simulink model "midterm_sim"  (R2022b)
settings: Solver=VariableStepAuto  StartTime=0.0  StopTime=Tf  RelTol=1e-3
undefined symbols (not defined in the file): h0, J, kd_nonlin, kp_nonlin, mu, q_inertial2body_0, q_inertial2LVLH_0, q_LVLH2body_0, q_LVLH2body_f, r_inertial_0, rate_max, Tf_man, use_CMG, v_inertial_0, w_b_LVLH_man, w_body_wrt_inertial_0, w_LVLH_wrt_inertial_in_LVLH
libraries: matrix_library x2
settings Model: Creator=corey  LastModifiedBy=corey
settings DebuggingCC: UnconnectedInputMsg=warning  UnconnectedOutputMsg=warning  UnconnectedLineMsg=warning
settings ModelReferenceCC: EnableRefExpFcnMdlSchedulingChecks=on
settings RTWCC: DLArmComputeVersion=19.05

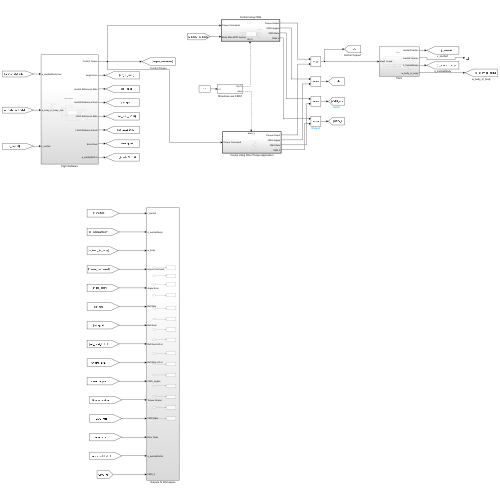
[thumbnail: Simulink's stored preview of the top-level diagram]
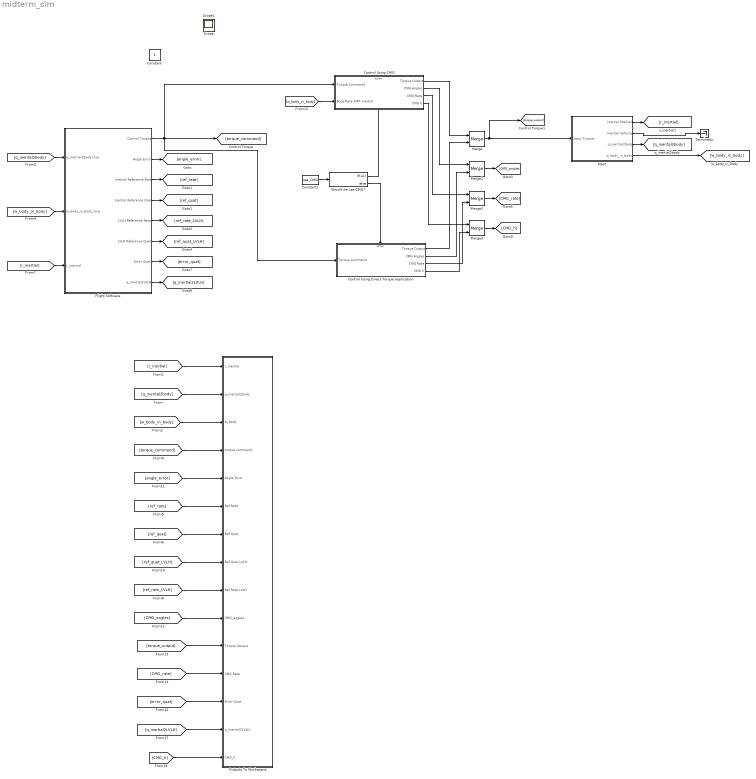
== system midterm_sim ==
  Constant1 : Constant  Value=use_CMG
  Control Using CMG : Subsystem  TreatAsAtomicUnit=on
  Control Using Direct Torque Application : Subsystem  TreatAsAtomicUnit=on
  Flight Software : Subsystem
  Merge{,1..3} (4 alike) : Merge
  Outputs To Workspace : Subsystem
  Plant : Subsystem
  Should we use CMG? : If  IfExpression=u1
  Terminator : Terminator
  Constant : Constant  IOType=siggen
  Scope : Scope
  Scope1 : Scope
  wires:
  Plant/4(w_body_in_body) -> [w_body_in_body]
  Plant/3(q_inertial2body) -> [q_inerital2body]
  Plant/2(Inertial Velocity) -> Terminator/1
  Plant/1(Inertial Position) -> [r_inertial]
  [q_inerital2body] -> Outputs To Workspace/2(q_inertial2body)
  [w_body_in_body] -> Outputs To Workspace/3(w_body)
  [r_inertial] -> Outputs To Workspace/1(r_inertial)
  [torque_command] -> Outputs To Workspace/4(torque command)
  Flight Software/1(Control Torque) -> Control Using CMG/1(Torque Command), Control Using Direct Torque Application/1(Torque Command), [torque_command]
  [angle_error] -> Outputs To Workspace/5(Angle Error)
  Flight Software/2(Angle Error) -> [angle_error]
  [q_inerital2body] -> Flight Software/1(q_inertial2body true)
  [w_body_in_body] -> Flight Software/2(w_body_in_body_true)
  Flight Software/3(Inertial Reference Rate) -> [ref_rate]
  Flight Software/4(Inertial Reference Quat) -> [ref_quat]
  [ref_rate] -> Outputs To Workspace/6(Ref Rate)
  [ref_quat] -> Outputs To Workspace/7(Ref Quat)
  [ref_rate_LVLH] -> Outputs To Workspace/9(Ref Rate LVLH)
  [ref_quat_LVLH] -> Outputs To Workspace/8(Ref Quat LVLH)
  Flight Software/5(LVLH Reference Rate) -> [ref_rate_LVLH]
  Flight Software/6(LVLH Reference Quat) -> [ref_quat_LVLH]
  [r_inertial] -> Flight Software/3(r_inertial)
  [CMG_angles] -> Outputs To Workspace/10(CMG_angles)
  [torque_output] -> Outputs To Workspace/11(Torque Output)
  [CMG_rate] -> Outputs To Workspace/12(CMG Rate)
  Constant1/1 -> Should we use CMG?/1
  Should we use CMG?/1 -> Control Using CMG/Action
  Should we use CMG?/2 -> Control Using Direct Torque Application/Action
  Control Using CMG/1(Torque Output) -> Merge/1
  Control Using Direct Torque Application/1(Torque Output) -> Merge/2
  Control Using CMG/2(CMG Angles) -> Merge1/1
  Control Using Direct Torque Application/2(CMG Angles) -> Merge1/2
  Control Using CMG/3(CMG Rate) -> Merge2/1
  Control Using Direct Torque Application/3(CMG Rate) -> Merge2/2
  Merge/1 -> Plant/1(Input Torque), [torque_output]
  Merge1/1 -> [CMG_angles]
  Merge2/1 -> [CMG_rate]
  [w_body_in_body] -> Control Using CMG/2(Body Rate WRT Inertial)
  Flight Software/7(Error Quat) -> [error_quat]
  [error_quat] -> Outputs To Workspace/13(Error Quat)
  Flight Software/8(q_inertial2LVLH) -> [q_inertial2LVLH]
  [q_inertial2LVLH] -> Outputs To Workspace/14(q_inertial2LVLH)
  Merge3/1 -> [CMG_h]
  Control Using CMG/4(CMG h) -> Merge3/1
  Control Using Direct Torque Application/4(CMG h) -> Merge3/2
  [CMG_h] -> Outputs To Workspace/15(CMG_h)

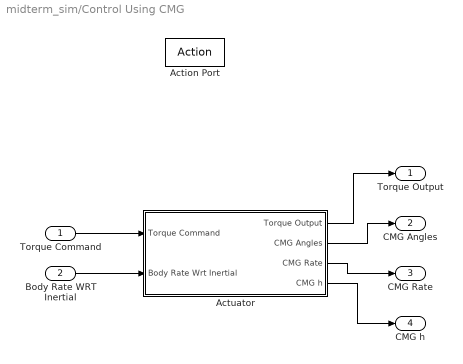
== system midterm_sim/Control Using CMG ==
  Torque Command : Inport
  Body Rate WRT Inertial : Inport  Port=2
  Action Port : ActionPort  ActionPortLabel=if(u1)
  Actuator : Subsystem
  Torque Output : Outport
  CMG Angles : Outport  Port=2
  CMG Rate : Outport  Port=3
  CMG h : Outport  Port=4
  wires:
  Torque Command/1 -> Actuator/1(Torque Command)
  Body Rate WRT Inertial/1 -> Actuator/2(Body Rate Wrt Inertial)
  Actuator/1(Torque Output) -> Torque Output/1
  Actuator/2(CMG Angles) -> CMG Angles/1
  Actuator/3(CMG Rate) -> CMG Rate/1
  Actuator/4(CMG h) -> CMG h/1

== system midterm_sim/Control Using Direct Torque Application ==
  Torque Command : Inport
  Action Port : ActionPort  ActionPortLabel=else
  Constant : Constant  Value=[0 0 0 0 0 0 0 0]'
  Constant1 : Constant  Value=[0 0 0]'
  Torque Output : Outport
  CMG Angles : Outport  Port=2
  CMG Rate : Outport  Port=3
  CMG h : Outport  Port=4
  wires:
  Constant/1 -> CMG Angles/1, CMG Rate/1
  Torque Command/1 -> Torque Output/1
  Constant1/1 -> CMG h/1

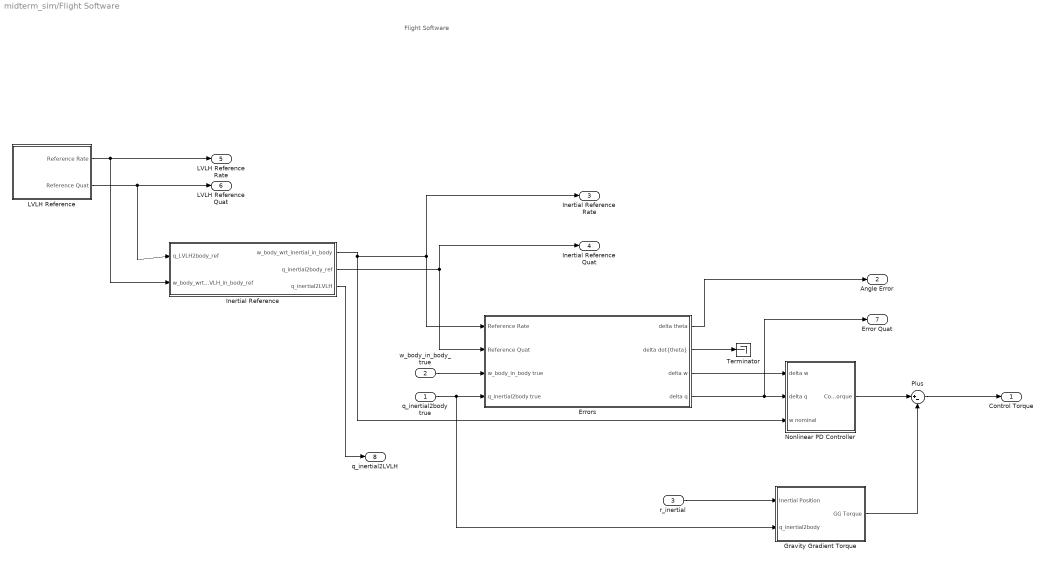
== system midterm_sim/Flight Software ==
  note: Flight Software
  q_inertial2body true : Inport
  w_body_in_body_true : Inport  Port=2
  r_inertial : Inport  Port=3
  Errors : Subsystem
  Gravity Gradient Torque : Subsystem
  Inertial Reference : Subsystem
  LVLH Reference : Subsystem
  Nonlinear PD Controller : Subsystem
  Plus : Sum  Inputs=|+-
  Terminator : Terminator
  Control Torque : Outport
  Angle Error : Outport  Port=2
  Inertial Reference Rate : Outport  Port=3
  Inertial Reference Quat : Outport  Port=4
  LVLH Reference Rate : Outport  Port=5
  LVLH Reference Quat : Outport  Port=6
  Error Quat : Outport  Port=7
  q_inertial2LVLH : Outport  Port=8
  wires:
  Errors/1(delta theta) -> Angle Error/1
  q_inertial2body true/1 -> Gravity Gradient Torque/2(q_inertial2body), Errors/4(q_inertial2body true)
  w_body_in_body_true/1 -> Errors/3(w_body_in_body true)
  Inertial Reference/1(w_body_wrt_inertial_in_body) -> Nonlinear PD Controller/3(w nominal), Inertial Reference Rate/1, Errors/1(Reference Rate)
  Inertial Reference/2(q_inertial2body_ref) -> Errors/2(Reference Quat), Inertial Reference Quat/1
  LVLH Reference/1(Reference Rate) -> Inertial Reference/2(w_body_wrt_LVLH_in_body_ref), LVLH Reference Rate/1
  LVLH Reference/2(Reference Quat) -> Inertial Reference/1(q_LVLH2body_ref), LVLH Reference Quat/1
  Errors/3(delta w) -> Nonlinear PD Controller/1(delta w)
  Errors/4(delta q) -> Error Quat/1, Nonlinear PD Controller/2(delta q)
  Errors/2("delta dot{theta}") -> Terminator/1
  Nonlinear PD Controller/1(Control Torque) -> Plus/1
  Plus/1 -> Control Torque/1
  Gravity Gradient Torque/1(GG Torque) -> Plus/2
  r_inertial/1 -> Gravity Gradient Torque/1(Inertial Position)
  Inertial Reference/3(q_inertial2LVLH) -> q_inertial2LVLH/1

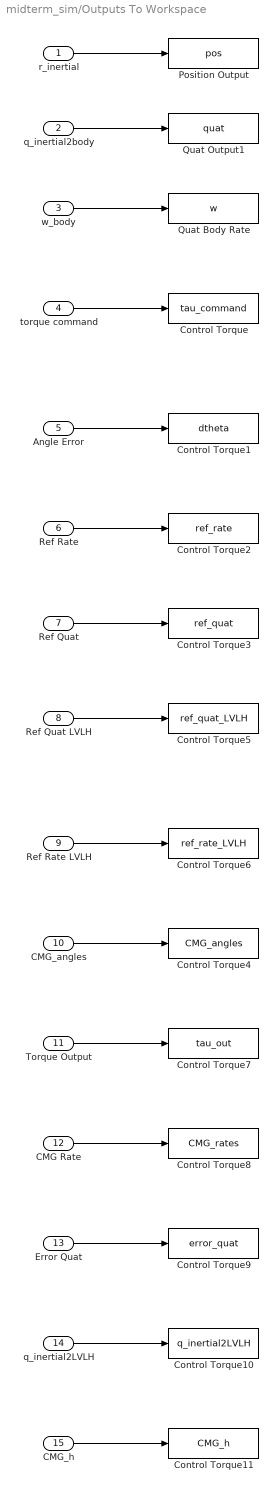
== system midterm_sim/Outputs To Workspace ==
  r_inertial : Inport
  q_inertial2body : Inport  Port=2
  w_body : Inport  Port=3
  torque command : Inport  Port=4
  Angle Error : Inport  Port=5
  Ref Rate : Inport  Port=6
  Ref Quat : Inport  Port=7
  Ref Quat LVLH : Inport  Port=8
  Ref Rate LVLH : Inport  Port=9
  CMG_angles : Inport  Port=10
  Torque Output : Inport  Port=11
  CMG Rate : Inport  Port=12
  Error Quat : Inport  Port=13
  q_inertial2LVLH : Inport  Port=14
  CMG_h : Inport  Port=15
  Control Torque : ToWorkspace  VariableName=tau_command  SampleTime=-1
  Control Torque1 : ToWorkspace  VariableName=dtheta  SampleTime=-1
  Control Torque10 : ToWorkspace  VariableName=q_inertial2LVLH  SampleTime=-1
  Control Torque11 : ToWorkspace  VariableName=CMG_h  SampleTime=-1
  Control Torque2 : ToWorkspace  VariableName=ref_rate  SampleTime=-1
  Control Torque3 : ToWorkspace  VariableName=ref_quat  SampleTime=-1
  Control Torque4 : ToWorkspace  VariableName=CMG_angles  SampleTime=-1
  Control Torque5 : ToWorkspace  VariableName=ref_quat_LVLH  SampleTime=-1
  Control Torque6 : ToWorkspace  VariableName=ref_rate_LVLH  SampleTime=-1
  Control Torque7 : ToWorkspace  VariableName=tau_out  SampleTime=-1
  Control Torque8 : ToWorkspace  VariableName=CMG_rates  SampleTime=-1
  Control Torque9 : ToWorkspace  VariableName=error_quat  SampleTime=-1
  Position Output : ToWorkspace  VariableName=pos  SampleTime=-1
  Quat Body Rate : ToWorkspace  VariableName=w  SampleTime=-1
  Quat Output1 : ToWorkspace  VariableName=quat  SampleTime=-1
  wires:
  r_inertial/1 -> Position Output/1
  w_body/1 -> Quat Body Rate/1
  q_inertial2body/1 -> Quat Output1/1
  torque command/1 -> Control Torque/1
  Angle Error/1 -> Control Torque1/1
  Ref Rate/1 -> Control Torque2/1
  Ref Quat/1 -> Control Torque3/1
  Ref Quat LVLH/1 -> Control Torque5/1
  Ref Rate LVLH/1 -> Control Torque6/1
  CMG_angles/1 -> Control Torque4/1
  Torque Output/1 -> Control Torque7/1
  CMG Rate/1 -> Control Torque8/1
  Error Quat/1 -> Control Torque9/1
  q_inertial2LVLH/1 -> Control Torque10/1
  CMG_h/1 -> Control Torque11/1

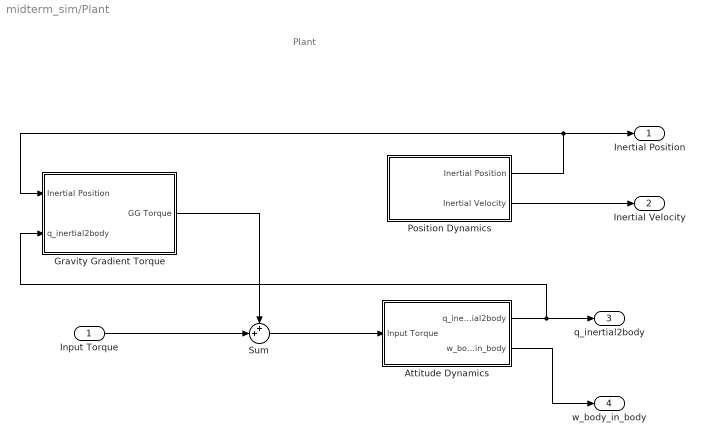
== system midterm_sim/Plant ==
  note: Plant
  Input Torque : Inport
  Attitude Dynamics : Subsystem
  Gravity Gradient Torque : Subsystem
  Position Dynamics : Subsystem
  Sum : Sum  Inputs=++|
  Inertial Position : Outport
  Inertial Velocity : Outport  Port=2
  q_inertial2body : Outport  Port=3
  w_body_in_body : Outport  Port=4
  wires:
  Position Dynamics/1(Inertial Position) -> Gravity Gradient Torque/1(Inertial Position), Inertial Position/1
  Position Dynamics/2(Inertial Velocity) -> Inertial Velocity/1
  Attitude Dynamics/1(q_inertial2body) -> Gravity Gradient Torque/2(q_inertial2body), q_inertial2body/1
  Attitude Dynamics/2(w_body_in_body) -> w_body_in_body/1
  Input Torque/1 -> Sum/2
  Sum/1 -> Attitude Dynamics/1(Input Torque)
  Gravity Gradient Torque/1(GG Torque) -> Sum/1

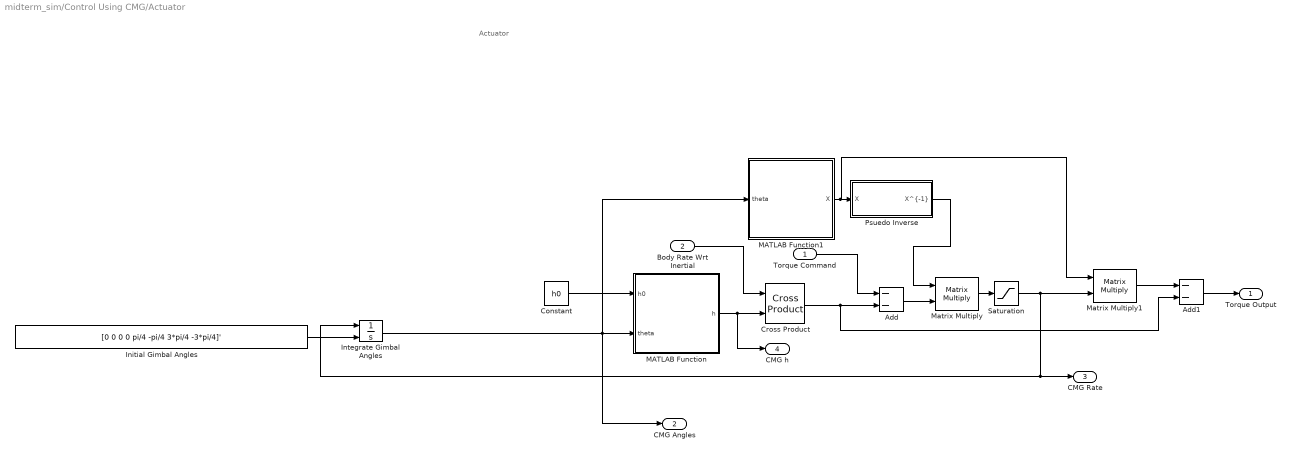
== system midterm_sim/Control Using CMG/Actuator ==
  note: Actuator
  Torque Command : Inport
  Body Rate Wrt Inertial : Inport  Port=2
  Add : Sum  Inputs=--
  Add1 : Sum  Inputs=--
  Constant : Constant  Value=h0
  Cross Product : matrix_library/Cross Product
  Initial Gimbal Angles : Constant  Value=[0 0 0 0 pi/4 -pi/4 3*pi/4 -3*pi/4]'
  Integrate Gimbal Angles : Integrator  InitialConditionSource=external
  MATLAB Function : MATLAB Function  TreatAsAtomicUnit=on
  MATLAB Function1 : MATLAB Function  TreatAsAtomicUnit=on
  Matrix Multiply : Product  Multiplication=Matrix(*)
  Matrix Multiply1 : Product  Multiplication=Matrix(*)
  Psuedo Inverse : Subsystem
  Saturation : Saturate  UpperLimit=rate_max  LowerLimit=-1*rate_max
  Torque Output : Outport
  CMG Angles : Outport  Port=2
  CMG Rate : Outport  Port=3
  CMG h : Outport  Port=4
  wires:
  Initial Gimbal Angles/1 -> Integrate Gimbal Angles/2
  Constant/1 -> MATLAB Function/1(h0)
  Cross Product/1 -> Add1/2, Add/2
  Torque Command/1 -> Add/1
  Body Rate Wrt Inertial/1 -> Cross Product/1
  MATLAB Function/1(h) -> CMG h/1, Cross Product/2
  MATLAB Function1/1(X) -> Matrix Multiply1/1, Psuedo Inverse/1(X)
  Psuedo Inverse/1("X^{-1}") -> Matrix Multiply/1
  Add/1 -> Matrix Multiply/2
  Matrix Multiply1/1 -> Add1/1
  Add1/1 -> Torque Output/1
  Integrate Gimbal Angles/1 -> MATLAB Function/2(theta), CMG Angles/1, MATLAB Function1/1(theta)
  Matrix Multiply/1 -> Saturation/1
  Saturation/1 -> Integrate Gimbal Angles/1, CMG Rate/1, Matrix Multiply1/2

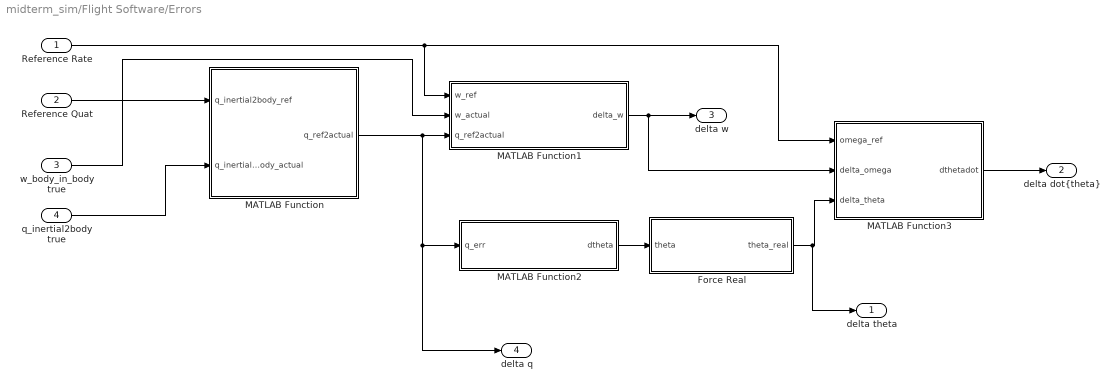
== system midterm_sim/Flight Software/Errors ==
  Reference Rate : Inport
  Reference Quat : Inport  Port=2
  w_body_in_body true : Inport  Port=3
  q_inertial2body true : Inport  Port=4
  Force Real : MATLAB Function  TreatAsAtomicUnit=on
  MATLAB Function : MATLAB Function  TreatAsAtomicUnit=on
  MATLAB Function1 : MATLAB Function  TreatAsAtomicUnit=on
  MATLAB Function2 : MATLAB Function  TreatAsAtomicUnit=on
  MATLAB Function3 : MATLAB Function  TreatAsAtomicUnit=on
  delta theta : Outport
  "delta dot{theta}" : Outport  Port=2
  delta w : Outport  Port=3
  delta q : Outport  Port=4
  wires:
  Reference Quat/1 -> MATLAB Function/1(q_inertial2body_ref)
  q_inertial2body true/1 -> MATLAB Function/2(q_inertial2body_actual)
  MATLAB Function/1(q_ref2actual) -> delta q/1, MATLAB Function2/1(q_err), MATLAB Function1/3(q_ref2actual)
  Reference Rate/1 -> MATLAB Function3/1(omega_ref), MATLAB Function1/1(w_ref)
  w_body_in_body true/1 -> MATLAB Function1/2(w_actual)
  MATLAB Function3/1(dthetadot) -> "delta dot{theta}"/1
  MATLAB Function2/1(dtheta) -> Force Real/1(theta)
  Force Real/1(theta_real) -> delta theta/1, MATLAB Function3/3(delta_theta)
  MATLAB Function1/1(delta_w) -> delta w/1, MATLAB Function3/2(delta_omega)

== system midterm_sim/Flight Software/Gravity Gradient Torque ==
  Inertial Position : Inport
  q_inertial2body : Inport  Port=2
  GG Torque Computation : MATLAB Function  TreatAsAtomicUnit=on
  Gravity Constant : Constant  Value=mu
  Inerita Matrix : Constant  Value=J
  MATLAB Function : MATLAB Function  TreatAsAtomicUnit=on
  GG Torque : Outport
  wires:
  Inerita Matrix/1 -> GG Torque Computation/1(J)
  Inertial Position/1 -> MATLAB Function/2(r), GG Torque Computation/3(r_inertial)
  q_inertial2body/1 -> GG Torque Computation/4(q_inertial2body)
  GG Torque Computation/1(T) -> GG Torque/1
  Gravity Constant/1 -> MATLAB Function/1(mu)
  MATLAB Function/1(n) -> GG Torque Computation/2(n)

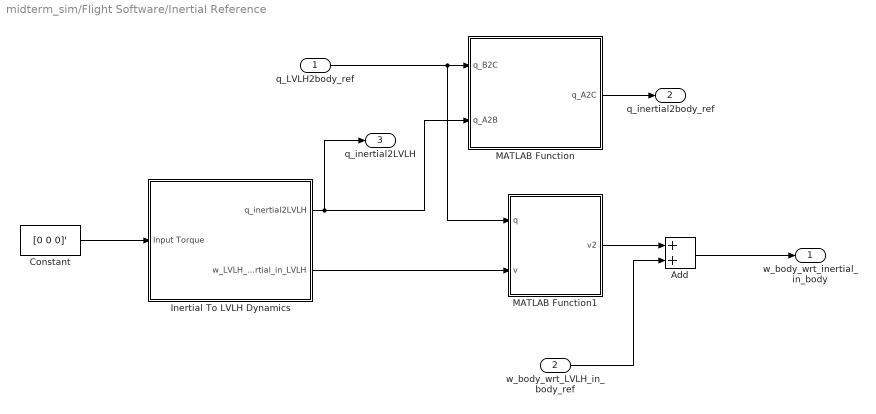
== system midterm_sim/Flight Software/Inertial Reference ==
  q_LVLH2body_ref : Inport
  w_body_wrt_LVLH_in_body_ref : Inport  Port=2
  Add : Sum
  Constant : Constant  Value=[0 0 0]'
  Inertial To LVLH Dynamics : Subsystem
  MATLAB Function : MATLAB Function  TreatAsAtomicUnit=on
  MATLAB Function1 : MATLAB Function  TreatAsAtomicUnit=on
  w_body_wrt_inertial_in_body : Outport
  q_inertial2body_ref : Outport  Port=2
  q_inertial2LVLH : Outport  Port=3
  wires:
  Constant/1 -> Inertial To LVLH Dynamics/1(Input Torque)
  Inertial To LVLH Dynamics/1(q_inertial2LVLH) -> MATLAB Function/2(q_A2B), q_inertial2LVLH/1
  MATLAB Function/1(q_A2C) -> q_inertial2body_ref/1
  q_LVLH2body_ref/1 -> MATLAB Function1/1(q), MATLAB Function/1(q_B2C)
  Inertial To LVLH Dynamics/2(w_LVLH_wrt_inertial_in_LVLH) -> MATLAB Function1/2(v)
  MATLAB Function1/1(v2) -> Add/1
  Add/1 -> w_body_wrt_inertial_in_body/1
  w_body_wrt_LVLH_in_body_ref/1 -> Add/2

== system midterm_sim/Flight Software/LVLH Reference ==
  Attitude Hold : Subsystem  TreatAsAtomicUnit=on
  Attitude Slew : Subsystem  TreatAsAtomicUnit=on
  Clock : Clock
  If : If  IfExpression=u1 < Tf_man
  Merge : Merge
  Merge1 : Merge
  Reference Rate : Outport
  Reference Quat : Outport  Port=2
  wires:
  Clock/1 -> If/1
  If/1 -> Attitude Slew/Action
  If/2 -> Attitude Hold/Action
  Attitude Slew/1(q_LVLH2body) -> Merge/1
  Attitude Hold/1(q_inertial2body) -> Merge/2
  Merge/1 -> Reference Quat/1
  Merge1/1 -> Reference Rate/1
  Attitude Slew/2(w_body_in_body) -> Merge1/1
  Attitude Hold/2(w_body) -> Merge1/2

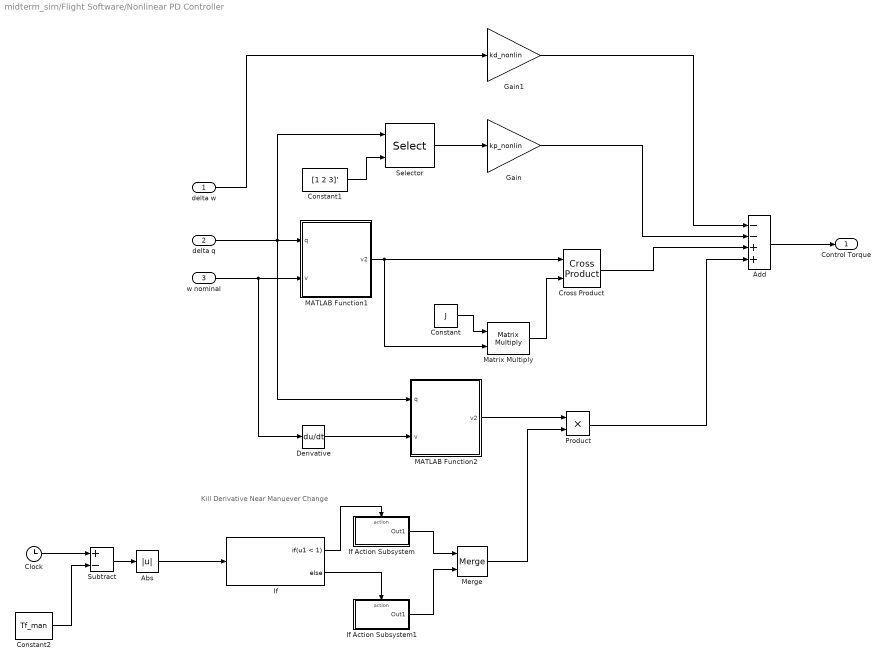
== system midterm_sim/Flight Software/Nonlinear PD Controller ==
  note: Kill Derivative Near Manuever Change
  delta w : Inport
  delta q : Inport  Port=2
  w nominal : Inport  Port=3
  Abs : Abs  SaturateOnIntegerOverflow=off
  Add : Sum  Inputs=--++
  Clock : Clock
  Constant : Constant  Value=J
  Constant1 : Constant  Value=[1 2 3]'
  Constant2 : Constant  Value=Tf_man
  Cross Product : matrix_library/Cross Product
  Derivative : Derivative  CoefficientInTFapproximation=Inf
  Gain : Gain  Gain=kp_nonlin
  Gain1 : Gain  Gain=kd_nonlin
  If : If  IfExpression=u1 < 1
  If Action Subsystem : Subsystem  TreatAsAtomicUnit=on
  If Action Subsystem1 : Subsystem  TreatAsAtomicUnit=on
  MATLAB Function1 : MATLAB Function  TreatAsAtomicUnit=on
  MATLAB Function2 : MATLAB Function  TreatAsAtomicUnit=on
  Matrix Multiply : Product  Multiplication=Matrix(*)
  Merge : Merge
  Product : Product
  Selector : Selector  InputPortWidth=4  IndexOptions=Index vector (port)  Indices=[1 3]  OutputSizes=1
  Subtract : Sum  Inputs=+-
  Control Torque : Outport
  wires:
  delta q/1 -> Selector/1, MATLAB Function2/1(q), MATLAB Function1/1(q)
  w nominal/1 -> Derivative/1, MATLAB Function1/2(v)
  MATLAB Function1/1(v2) -> Matrix Multiply/2, Cross Product/1
  Constant/1 -> Matrix Multiply/1
  Matrix Multiply/1 -> Cross Product/2
  Derivative/1 -> MATLAB Function2/2(v)
  Add/1 -> Control Torque/1
  Constant1/1 -> Selector/2
  Selector/1 -> Gain/1
  Gain/1 -> Add/2
  delta w/1 -> Gain1/1
  Gain1/1 -> Add/1
  MATLAB Function2/1(v2) -> Product/1
  Product/1 -> Add/4
  Cross Product/1 -> Add/3
  If/1 -> If Action Subsystem/Action
  If/2 -> If Action Subsystem1/Action
  Clock/1 -> Subtract/1
  Constant2/1 -> Subtract/2
  Subtract/1 -> Abs/1
  Abs/1 -> If/1
  If Action Subsystem/1(Out1) -> Merge/1
  If Action Subsystem1/1(Out1) -> Merge/2
  Merge/1 -> Product/2

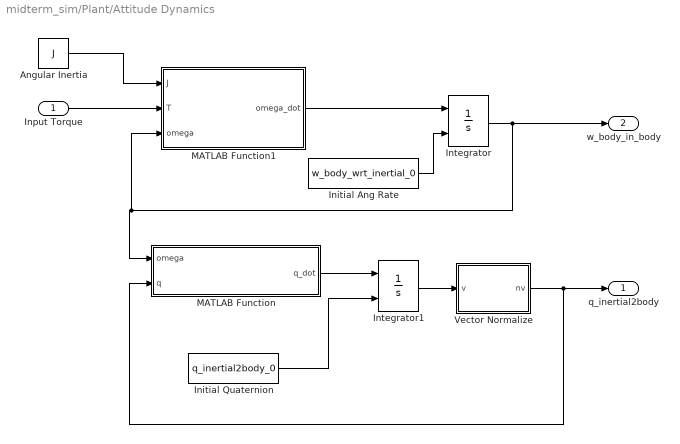
== system midterm_sim/Plant/Attitude Dynamics ==
  Input Torque : Inport
  Angular Inertia : Constant  Value=J
  Initial Ang Rate : Constant  Value=w_body_wrt_inertial_0
  Initial Quaternion : Constant  Value=q_inertial2body_0
  Integrator : Integrator  InitialConditionSource=external
  Integrator1 : Integrator  InitialConditionSource=external
  MATLAB Function : MATLAB Function  TreatAsAtomicUnit=on
  MATLAB Function1 : MATLAB Function  TreatAsAtomicUnit=on
  Vector Normalize : MATLAB Function  TreatAsAtomicUnit=on
  q_inertial2body : Outport
  w_body_in_body : Outport  Port=2
  wires:
  Integrator/1 -> MATLAB Function1/3(omega), MATLAB Function/1(omega), w_body_in_body/1
  MATLAB Function1/1(omega_dot) -> Integrator/1
  Initial Ang Rate/1 -> Integrator/2
  MATLAB Function/1(q_dot) -> Integrator1/1
  Initial Quaternion/1 -> Integrator1/2
  Integrator1/1 -> Vector Normalize/1(v)
  Vector Normalize/1(nv) -> MATLAB Function/2(q), q_inertial2body/1
  Input Torque/1 -> MATLAB Function1/2(T)
  Angular Inertia/1 -> MATLAB Function1/1(J)

== system midterm_sim/Plant/Gravity Gradient Torque ==
  Inertial Position : Inport
  q_inertial2body : Inport  Port=2
  GG Torque Computation : MATLAB Function  TreatAsAtomicUnit=on
  Gravity Constant : Constant  Value=mu
  Inerita Matrix : Constant  Value=J
  MATLAB Function : MATLAB Function  TreatAsAtomicUnit=on
  GG Torque : Outport
  wires:
  Inerita Matrix/1 -> GG Torque Computation/1(J)
  Inertial Position/1 -> MATLAB Function/2(r), GG Torque Computation/3(r_inertial)
  q_inertial2body/1 -> GG Torque Computation/4(q_inertial2body)
  GG Torque Computation/1(T) -> GG Torque/1
  Gravity Constant/1 -> MATLAB Function/1(mu)
  MATLAB Function/1(n) -> GG Torque Computation/2(n)

== system midterm_sim/Plant/Position Dynamics ==
  Gravity Constant : Constant  Value=mu
  Initial Position : Constant  Value=r_inertial_0
  Initial Velocity : Constant  Value=v_inertial_0
  Integrator : Integrator  InitialConditionSource=external  InitialCondition=[6871, 0, 0]'
  Integrator1 : Integrator  InitialConditionSource=external  InitialCondition=[0, 7.6166, 0]'
  Vector Norm : MATLAB Function  TreatAsAtomicUnit=on
  Inertial Position : Outport
  Inertial Velocity : Outport  Port=2
  wires:
  Integrator/1 -> Vector Norm/1(r), Inertial Position/1  "Position"
  Integrator1/1 -> Inertial Velocity/1, Integrator/1  "Velocity"
  Vector Norm/1(a) -> Integrator1/1  "Accel"
  Gravity Constant/1 -> Vector Norm/2(mu)
  Initial Velocity/1 -> Integrator1/2
  Initial Position/1 -> Integrator/2

== system midterm_sim/Control Using CMG/Actuator/Psuedo Inverse ==
  X : Inport
  Matrix Divide : Product  Inputs=*/  Multiplication=Matrix(*)
  Matrix Multiply : Product  Multiplication=Matrix(*)
  Transpose : Math  Operator=transpose
  "X^{-1}" : Outport
  wires:
  Transpose/1 -> Matrix Divide/1, Matrix Multiply/2
  X/1 -> Transpose/1, Matrix Multiply/1
  Matrix Multiply/1 -> Matrix Divide/2
  Matrix Divide/1 -> "X^{-1}"/1

== system midterm_sim/Flight Software/Inertial Reference/Inertial To LVLH Dynamics ==
  Input Torque : Inport
  Attitude Dynamics : Subsystem
  q_inertial2LVLH : Outport
  w_LVLH_wrt_inertial_in_LVLH : Outport  Port=2
  wires:
  Input Torque/1 -> Attitude Dynamics/1(Input Torque)
  Attitude Dynamics/1(q_LVLH2body) -> q_inertial2LVLH/1
  Attitude Dynamics/2(w_body_in_body) -> w_LVLH_wrt_inertial_in_LVLH/1

== system midterm_sim/Flight Software/LVLH Reference/Attitude Hold ==
  Action Port : ActionPort  ActionPortLabel=else
  Constant : Constant  Value=q_LVLH2body_f
  Constant1 : Constant  Value=[0 0 0]'
  q_inertial2body : Outport
  w_body : Outport  Port=2
  wires:
  Constant/1 -> q_inertial2body/1
  Constant1/1 -> w_body/1

== system midterm_sim/Flight Software/LVLH Reference/Attitude Slew ==
  Action Port : ActionPort  ActionPortLabel=if(u1 < Tf_man)
  Constant : Constant  Value=[0 0 0]'
  Reference Plant : Subsystem
  q_LVLH2body : Outport
  w_body_in_body : Outport  Port=2
  wires:
  Constant/1 -> Reference Plant/1(Input Torque)
  Reference Plant/1(q_inertial2body) -> q_LVLH2body/1
  Reference Plant/2(w_body_in_body) -> w_body_in_body/1

== system midterm_sim/Flight Software/Nonlinear PD Controller/If Action Subsystem ==
  Action Port : ActionPort  ActionPortLabel=if(u1 < 1)
  Constant : Constant  Value=0
  Out1 : Outport
  wires:
  Constant/1 -> Out1/1

== system midterm_sim/Flight Software/Nonlinear PD Controller/If Action Subsystem1 ==
  Action Port : ActionPort  ActionPortLabel=else
  Constant : Constant
  Out1 : Outport
  wires:
  Constant/1 -> Out1/1

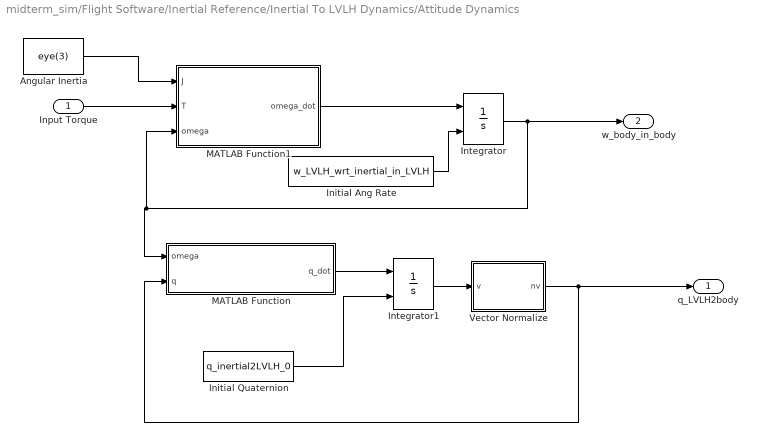
== system midterm_sim/Flight Software/Inertial Reference/Inertial To LVLH Dynamics/Attitude Dynamics ==
  Input Torque : Inport
  Angular Inertia : Constant  Value=eye(3)
  Initial Ang Rate : Constant  Value=w_LVLH_wrt_inertial_in_LVLH
  Initial Quaternion : Constant  Value=q_inertial2LVLH_0
  Integrator : Integrator  InitialConditionSource=external
  Integrator1 : Integrator  InitialConditionSource=external
  MATLAB Function : MATLAB Function  TreatAsAtomicUnit=on
  MATLAB Function1 : MATLAB Function  TreatAsAtomicUnit=on
  Vector Normalize : MATLAB Function  TreatAsAtomicUnit=on
  q_LVLH2body : Outport
  w_body_in_body : Outport  Port=2
  wires:
  Integrator/1 -> MATLAB Function1/3(omega), MATLAB Function/1(omega), w_body_in_body/1
  MATLAB Function1/1(omega_dot) -> Integrator/1
  Initial Ang Rate/1 -> Integrator/2
  MATLAB Function/1(q_dot) -> Integrator1/1
  Initial Quaternion/1 -> Integrator1/2
  Integrator1/1 -> Vector Normalize/1(v)
  Vector Normalize/1(nv) -> q_LVLH2body/1, MATLAB Function/2(q)
  Input Torque/1 -> MATLAB Function1/2(T)
  Angular Inertia/1 -> MATLAB Function1/1(J)

== system midterm_sim/Flight Software/LVLH Reference/Attitude Slew/Reference Plant ==
  Input Torque : Inport
  Attitude Dynamics : Subsystem
  q_inertial2body : Outport
  w_body_in_body : Outport  Port=2
  wires:
  Input Torque/1 -> Attitude Dynamics/1(Input Torque)
  Attitude Dynamics/1(q_LVLH2body) -> q_inertial2body/1
  Attitude Dynamics/2(w_body_in_body) -> w_body_in_body/1

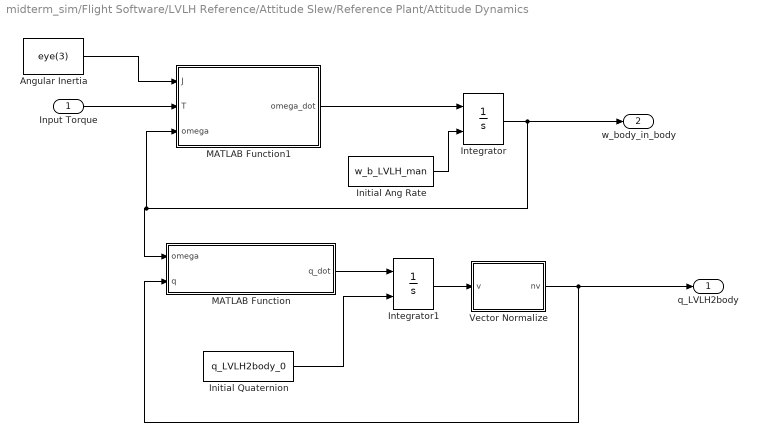
== system midterm_sim/Flight Software/LVLH Reference/Attitude Slew/Reference Plant/Attitude Dynamics ==
  Input Torque : Inport
  Angular Inertia : Constant  Value=eye(3)
  Initial Ang Rate : Constant  Value=w_b_LVLH_man
  Initial Quaternion : Constant  Value=q_LVLH2body_0
  Integrator : Integrator  InitialConditionSource=external
  Integrator1 : Integrator  InitialConditionSource=external
  MATLAB Function : MATLAB Function  TreatAsAtomicUnit=on
  MATLAB Function1 : MATLAB Function  TreatAsAtomicUnit=on
  Vector Normalize : MATLAB Function  TreatAsAtomicUnit=on
  q_LVLH2body : Outport
  w_body_in_body : Outport  Port=2
  wires:
  Integrator/1 -> MATLAB Function1/3(omega), MATLAB Function/1(omega), w_body_in_body/1
  MATLAB Function1/1(omega_dot) -> Integrator/1
  Initial Ang Rate/1 -> Integrator/2
  MATLAB Function/1(q_dot) -> Integrator1/1
  Initial Quaternion/1 -> Integrator1/2
  Integrator1/1 -> Vector Normalize/1(v)
  Vector Normalize/1(nv) -> q_LVLH2body/1, MATLAB Function/2(q)
  Input Torque/1 -> MATLAB Function1/2(T)
  Angular Inertia/1 -> MATLAB Function1/1(J)

== matlab function midterm_sim/Plant/Attitude Dynamics/MATLAB Function ==
  data: omega input; q_dot output; q input
function q_dot = QuaternionEvolution(omega, q)
intermed = [omega; 0];
q_dot = 0.5*QuatProduct(intermed,q);

== matlab function midterm_sim/Flight Software/LVLH Reference/Attitude Slew/Reference Plant/Attitude Dynamics/MATLAB Function ==
  data: omega input; q_dot output; q input
function q_dot = QuaternionEvolution(omega, q)
intermed = [omega; 0];
q_dot = 0.5*QuatProduct(intermed,q);

== matlab function midterm_sim/Flight Software/LVLH Reference/Attitude Slew/Reference Plant/Attitude Dynamics/MATLAB Function1 ==
  data: J input; omega_dot output; T input; omega input
function omega_dot = OmegaEvolution(J, T, omega)
omega_dot = J\(T - cross(omega, J*omega));

== matlab function midterm_sim/Flight Software/LVLH Reference/Attitude Slew/Reference Plant/Attitude Dynamics/Vector Normalize ==
  data: v input; nv output
function nv = NormVec(v)

nv = v/norm(v);

== matlab function midterm_sim/Flight Software/Nonlinear PD Controller/MATLAB Function1 ==
  data: q input; v2 output; v input
function v2 = QuatRotate_sym(q,v)

v2 = QuatTransform(q,v);

== matlab function midterm_sim/Flight Software/Errors/Force Real ==
  data: theta input; theta_real output
function theta_real = ForceReal(theta)

theta_real = real(theta);

== matlab function midterm_sim/Flight Software/Inertial Reference/MATLAB Function1 ==
  data: q input; v2 output; v input
function v2 = QuatRotate_sym(q,v)

v2 = QuatTransform(q,v);

== matlab function midterm_sim/Flight Software/Nonlinear PD Controller/MATLAB Function2 ==
  data: q input; v2 output; v input
function v2 = QuatRotate_sym(q,v)

v2 = QuatTransform(q,v);

== matlab function midterm_sim/Plant/Gravity Gradient Torque/GG Torque Computation ==
  data: J input; T output; n input; r_inertial input; q_inertial2body input
function T = GGTorque(J, n, r_inertial, q_inertial2body)

% Down in body frame
down_inertial = -r_inertial/norm(r_inertial);
down_body = QuatTransform(q_inertial2body,down_inertial);

% Gravity gradient torque
T = 3*n^2*cross(down_body,J*down_body);

== matlab function midterm_sim/Plant/Gravity Gradient Torque/MATLAB Function ==
  data: mu input; n output; r input
function n = OrbitRate(mu,r)

n = sqrt(mu/norm(r)^3);

== matlab function midterm_sim/Plant/Position Dynamics/Vector Norm ==
  data: r input; a output; mu input
function a = TwoBodyGrav(r,mu)

nr = norm(r);
a = -mu*r/(nr^3);

== matlab function midterm_sim/Flight Software/Gravity Gradient Torque/GG Torque Computation ==
  data: J input; T output; n input; r_inertial input; q_inertial2body input
function T = GGTorque(J, n, r_inertial, q_inertial2body)

% Down in body frame
down_inertial = -r_inertial/norm(r_inertial);
down_body = QuatTransform(q_inertial2body,down_inertial);

% Gravity gradient torque
T = 3*n^2*cross(down_body,J*down_body);

== matlab function midterm_sim/Flight Software/Gravity Gradient Torque/MATLAB Function ==
  data: mu input; n output; r input
function n = OrbitRate(mu,r)

n = sqrt(mu/norm(r)^3);

== matlab function midterm_sim/Control Using CMG/Actuator/MATLAB Function ==
  data: h0 input; h output; theta input
function h = CMG_AngMom(h0, theta)
% Produces the angular momentum vector for the CMGs

% Extract alpha and betas
alphas = theta(1:4);
betas = theta(5:8);

h = zeros(3,1);
for ii = 1:4
    h = h + h0*[sin(alphas(ii)); cos(alphas(ii))*cos(betas(ii)); cos(alphas(ii))*sin(betas(ii))];
end

== matlab function midterm_sim/Control Using CMG/Actuator/MATLAB Function1 ==
  data: X output; theta input
function X = CMG_X(theta)
% Produces the matrix of CMG spin axes

% Extract alpha and betas
alphas = theta(1:4);
betas = theta(5:8);

X = zeros(3,8);
for ii = 1:4
    X(:,2*ii-1:2*ii) = [cos(alphas(ii)), 0;
        -sin(alphas(ii))*cos(betas(ii)), -cos(alphas(ii))*sin(betas(ii));
        -sin(alphas(ii))*sin(betas(ii)), cos(alphas(ii))*cos(betas(ii))];
end

== matlab function midterm_sim/Plant/Attitude Dynamics/MATLAB Function1 ==
  data: J input; omega_dot output; T input; omega input
function omega_dot = OmegaEvolution(J, T, omega)
omega_dot = J\(T - cross(omega, J*omega));

== matlab function midterm_sim/Plant/Attitude Dynamics/Vector Normalize ==
  data: v input; nv output
function nv = NormVec(v)

nv = v/norm(v);

== matlab function midterm_sim/Flight Software/Inertial Reference/Inertial To LVLH Dynamics/Attitude Dynamics/MATLAB Function ==
  data: omega input; q_dot output; q input
function q_dot = QuaternionEvolution(omega, q)
intermed = [omega; 0];
q_dot = 0.5*QuatProduct(intermed,q);

== matlab function midterm_sim/Flight Software/Inertial Reference/Inertial To LVLH Dynamics/Attitude Dynamics/MATLAB Function1 ==
  data: J input; omega_dot output; T input; omega input
function omega_dot = OmegaEvolution(J, T, omega)
omega_dot = J\(T - cross(omega, J*omega));

== matlab function midterm_sim/Flight Software/Inertial Reference/Inertial To LVLH Dynamics/Attitude Dynamics/Vector Normalize ==
  data: v input; nv output
function nv = NormVec(v)

nv = v/norm(v);

== matlab function midterm_sim/Flight Software/Errors/MATLAB Function ==
  data: q_inertial2body_ref input; q_ref2actual output; q_inertial2body_actual input
function q_ref2actual = ErrorQuat(q_inertial2body_ref, q_inertial2body_actual)

q_ref2actual = QuatProduct(q_inertial2body_actual,QuatInv(q_inertial2body_ref));

% Force normalization
q_ref2actual = q_ref2actual/norm(q_ref2actual);

== matlab function midterm_sim/Flight Software/Errors/MATLAB Function1 ==
  data: w_ref input; delta_w output; w_actual input; q_ref2actual input
function delta_w = ErrorRate(w_ref, w_actual, q_ref2actual)

delta_w = w_actual - QuatTransform(q_ref2actual,w_ref);

== matlab function midterm_sim/Flight Software/Errors/MATLAB Function2 ==
  data: q_err input; dtheta output
function dtheta = ErrorQuat2ErrorAngle(q_err)

% Quaternion components
q_v = real(q_err(1:3));
q_s = real(q_err(4));

dtheta = [atan2(q_v(1),q_s);
    atan2(q_v(2),q_s);
    atan2(q_v(3),q_s)];

== matlab function midterm_sim/Flight Software/Errors/MATLAB Function3 ==
  data: omega_ref input; dthetadot output; delta_omega input; delta_theta input
function dthetadot = ErrorThetaDot(omega_ref, delta_omega, delta_theta)

dthetadot = delta_omega - cross(omega_ref,delta_theta);

== matlab function midterm_sim/Flight Software/Inertial Reference/MATLAB Function ==
  data: q_B2C input; q_A2C output; q_A2B input
function q_A2C = QuatProduct_sym(q_B2C,q_A2B)

q_A2C = QuatProduct(q_B2C,q_A2B);
